simulink model "Daolibai_design_SFandOFtu"  (R2016a)
settings: Solver=VariableStepAuto  SolverMode=SingleTasking  StartTime=0.0  StopTime=20.0  RelTol=1e-3
values from neighbouring files (symbols this model uses):
  A1 = [0 1 0 0 ... (first row only)    [Daolibai_analysis_ControllAndObserv.m]    (also in Daolibai_analysis_stability.m; Daolibai_design_OSF.m; Daolibai_design_OSFandPIOF.m = [A [0 0 0 0]'; Daolibai_design_SF.m)
  B1 = [0;1;0;-2]    [Daolibai_analysis_ControllAndObserv.m]    (also in Daolibai_analysis_stability.m; Daolibai_design_OSF.m; Daolibai_design_OSFandPIOF.m = [B;0]; Daolibai_design_SF.m)
  C = [1 0 0]    [Caishidianlu_design.m]    (also in Daolibai_analysis_ControllAndObserv.m = [1 0 0 0]; Daolibai_analysis_stability.m = [1 0 0 0]; Daolibai_design_OSF.m = [1 0 0 0]; Daolibai_design_OSFandPIOF.m = [1 0 0 0])
  Init = [0.1 0.1 0.5 0.5]    [Daolibai_design_OSF.m]    (also in Daolibai_design_OSFandPIOF.m = [0 0.04 0.005 0.1 ]; Daolibai_design_SFandOF.m; Daolibai_design_SFandPIOF.m = [0 0.1 0.005 0.1 ])
  K = inv(P1)*V1    [Caishidianlu_design.m]    (also in Daolibai_design_OSF.m = acker(A1,B1,P1); Daolibai_design_OSFandPIOF.m = acker(A1,B1,P); Daolibai_design_SF.m = acker(A1,B1,P); Daolibai_design_SFandOF.m = acker(A,B,P))
settings Model: Creator=19017  LastModifiedBy=19017
settings DataIOCC: ReturnWorkspaceOutputs=on
settings DebuggingCC: SFUnexpectedBacktrackingDiag=error  SFNoUnconditionalDefaultTransitionDiag=error
settings SFSimCC: SimUseLocalCustomCode=on
settings RTWCC: RTWUseLocalCustomCode=on
settings GRTTargetCC: TargetLangStandard=C99 (ISO)
settings ConfigComp: CovMetricSettings=dwe  CovSaveCumulativeToWorkspaceVar=off  CovSaveSingleToWorkspaceVar=off  CovExternalEMLEnable=on

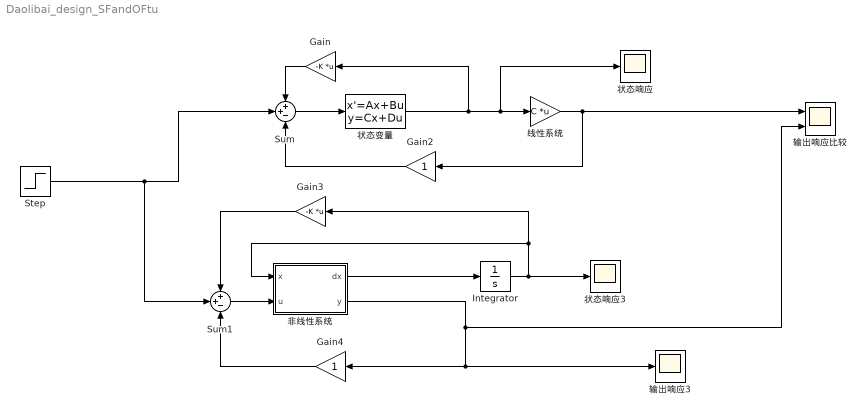
== system Daolibai_design_SFandOFtu ==
  Gain : Gain  Gain=-K  Multiplication=Matrix(K*u)
  Gain2 : Gain
  Gain3 : Gain  Gain=-K  Multiplication=Matrix(K*u)
  Gain4 : Gain
  Integrator : Integrator  InitialCondition=Init
  Step : Step  SampleTime=0
  Sum : Sum  Inputs=++-
  Sum1 : Sum  Inputs=++-
  状态变量 : StateSpace  A=A1  B=B1  C=eye(4)  D=[0;0;0;0]  X0=Init
  状态响应 : Scope
  状态响应3 : Scope
  线性系统 : Gain  Gain=C  Multiplication=Matrix(K*u)
  输出响应3 : Scope
  输出响应比较 : Scope  NumInputPorts=2
  非线性系统 : MATLAB Function  TreatAsAtomicUnit=on
  wires:
  线性系统/1 -> Gain2/1, 输出响应比较/1
  状态变量/1 -> Gain/1, 状态响应/1, 线性系统/1
  Sum/1 -> 状态变量/1
  Gain/1 -> Sum/1
  Gain2/1 -> Sum/3
  非线性系统/1(dx) -> Integrator/1
  Integrator/1 -> 状态响应3/1, Gain3/1, 非线性系统/1(x)
  非线性系统/2(y) -> 输出响应3/1, Gain4/1, 输出响应比较/2
  Sum1/1 -> 非线性系统/2(u)
  Gain3/1 -> Sum1/1
  Gain4/1 -> Sum1/3
  Step/1 -> Sum1/2, Sum/2

== matlab function Daolibai_design_SFandOFtu/非线性系统 ==
  data: x input; dx output; u input; y output
function [dx,y] = fcn(x,u)
dx = zeros(4,1);
M = 1;
m = 0.1;
l = 0.5;
g = 9.8;
dx(1) = x(2);
dx(2) = (u+m*l*x(4)^2*sin(x(3))-m*g*sin(x(3))*cos(x(3)))/(M+m-m*cos(x(3))^2);
dx(3) = x(4);
dx(4) = (-u*cos(x(3))+(M+m)*g*sin(x(3))-m*l*x(4)^2*sin(x(3))*cos(x(3)))/((M+m)*l-m*l*cos(x(3))^2);
y = x(1);
